simulink model "inertiaEstimation"  (R2024a)
settings: Solver=VariableStepAuto  StartTime=0.0  StopTime=1000  FixedStep=0.001  RelTol=1e-3
undefined symbols (not defined in the file or in its folder): esti, sat
settings Model: Creator=b_ant  LastModifiedBy=b_ant

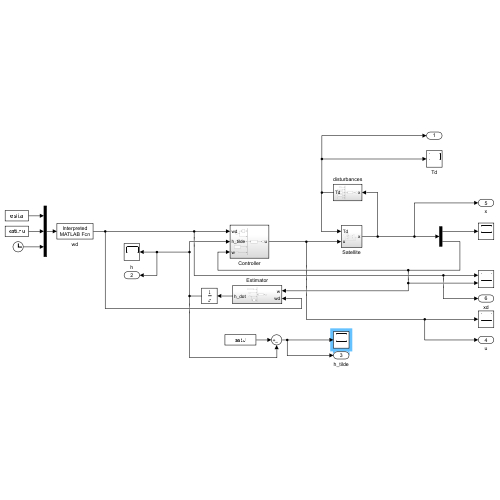
[thumbnail: Simulink's stored preview of the top-level diagram]
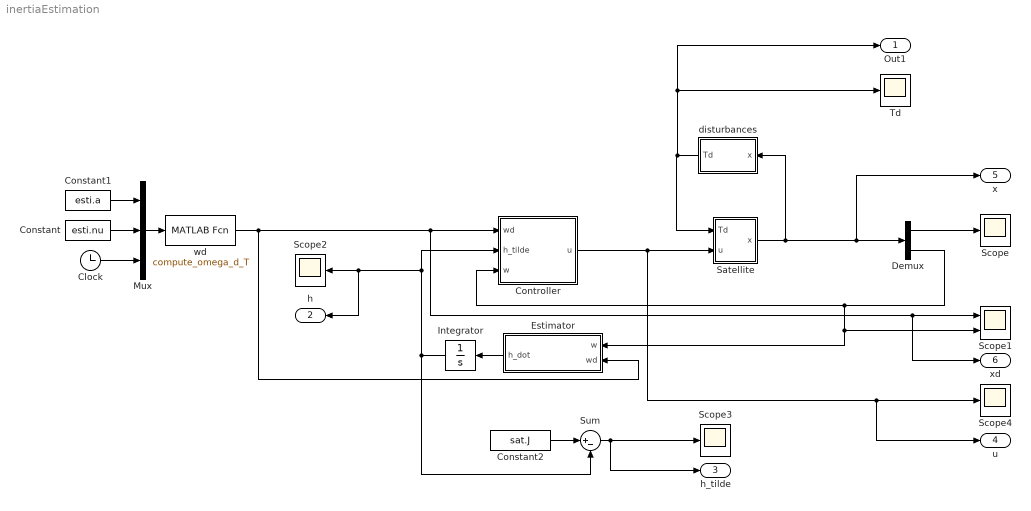
== system inertiaEstimation ==
  Clock : Clock
  Constant : Constant  Value=esti.nu
  Constant1 : Constant  Value=esti.a
  Constant2 : Constant  Value=sat.J
  Controller : Subsystem
  Demux : Demux  Outputs=2
  Estimator : Subsystem
  Integrator : Integrator
  Mux : Mux  Inputs=3
  Satellite : Subsystem
  Scope{,2..4} (4 alike) : Scope
  Scope1 : Scope  NumInputPorts=2
  Sum : Sum  Inputs=|+-
  Td : Scope
  disturbances : Subsystem
  wd : MATLABFcn  MATLABFcn=compute_omega_d_T
  Out1 : Outport
  h : Outport  Port=2
  h_tilde : Outport  Port=3
  u : Outport  Port=4
  x : Outport  Port=5
  xd : Outport  Port=6
  wires:
  Controller/1(u) -> u/1, Scope4/1, Satellite/2(u)
  Satellite/1(x) -> x/1, Demux/1, disturbances/1(x)
  wd/1 -> xd/1, Scope1/1, Controller/1(wd), Estimator/2(wd)
  Demux/2 -> Estimator/1(w), Scope1/2, Controller/3(w)
  Integrator/1 -> Controller/2(h_tilde), h/1, Scope2/1, Sum/2
  Estimator/1(h_dot) -> Integrator/1
  Demux/1 -> Scope/1
  Mux/1 -> wd/1
  Clock/1 -> Mux/3
  Constant/1 -> Mux/2
  Constant1/1 -> Mux/1
  Constant2/1 -> Sum/1
  Sum/1 -> h_tilde/1, Scope3/1
  disturbances/1(Td) -> Out1/1, Td/1, Satellite/1(Td)

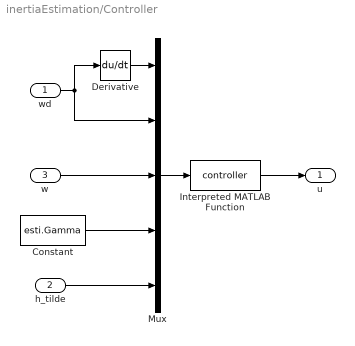
== system inertiaEstimation/Controller ==
  wd : Inport
  h_tilde : Inport  Port=2
  w : Inport  Port=3
  Constant : Constant  Value=esti.Gamma
  Derivative : Derivative
  Interpreted MATLAB Function : MATLABFcn  MATLABFcn=controller
  Mux : Mux  Inputs=5
  u : Outport
  wires:
  h_tilde/1 -> Mux/5
  w/1 -> Mux/3
  Constant/1 -> Mux/4
  Interpreted MATLAB Function/1 -> u/1
  Mux/1 -> Interpreted MATLAB Function/1
  wd/1 -> Mux/2, Derivative/1
  Derivative/1 -> Mux/1

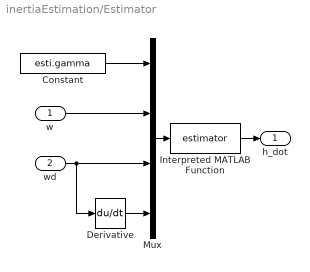
== system inertiaEstimation/Estimator ==
  w : Inport
  wd : Inport  Port=2
  Constant : Constant  Value=esti.gamma  VectorParams1D=off
  Derivative : Derivative
  Interpreted MATLAB Function : MATLABFcn  MATLABFcn=estimator
  Mux : Mux
  h_dot : Outport
  wires:
  Mux/1 -> Interpreted MATLAB Function/1
  Derivative/1 -> Mux/4
  wd/1 -> Derivative/1, Mux/3
  w/1 -> Mux/2
  Interpreted MATLAB Function/1 -> h_dot/1
  Constant/1 -> Mux/1

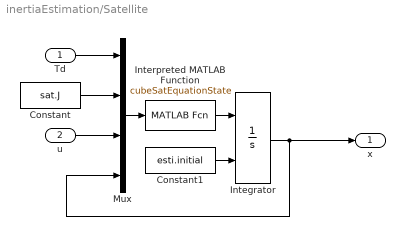
== system inertiaEstimation/Satellite ==
  Td : Inport
  u : Inport  Port=2
  Constant : Constant  Value=sat.J
  Constant1 : Constant  Value=esti.initial
  Integrator : Integrator  InitialConditionSource=external
  Interpreted MATLAB Function : MATLABFcn  MATLABFcn=cubeSatEquationState
  Mux : Mux
  x : Outport
  wires:
  u/1 -> Mux/3
  Integrator/1 -> x/1, Mux/4
  Mux/1 -> Interpreted MATLAB Function/1
  Interpreted MATLAB Function/1 -> Integrator/1
  Constant/1 -> Mux/2
  Td/1 -> Mux/1
  Constant1/1 -> Integrator/2

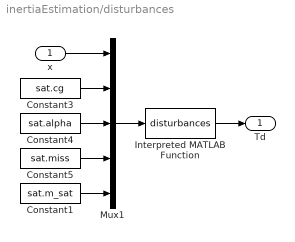
== system inertiaEstimation/disturbances ==
  x : Inport
  Constant1 : Constant  Value=sat.m_sat
  Constant3 : Constant  Value=sat.cg
  Constant4 : Constant  Value=sat.alpha
  Constant5 : Constant  Value=sat.miss
  Interpreted MATLAB Function : MATLABFcn  MATLABFcn=disturbances
  Mux1 : Mux  Inputs=5
  Td : Outport
  wires:
  Constant5/1 -> Mux1/4
  Constant3/1 -> Mux1/2
  Constant4/1 -> Mux1/3
  Mux1/1 -> Interpreted MATLAB Function/1
  Interpreted MATLAB Function/1 -> Td/1
  x/1 -> Mux1/1
  Constant1/1 -> Mux1/5
